simulink model "untitled3"  (Simulink 7.7)
settings: Solver=ode45  StartTime=0.0  StopTime=10.0  RelTol=1e-3
settings Model: Creator=güler  LastModifiedBy=güler

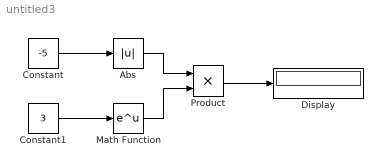
== system untitled3 ==
  Abs : Abs
  Constant : Constant  Value=-5
  Constant1 : Constant  Value=3
  Display : Display
  Math Function : Math  SaturateOnIntegerOverflow=on
  Product : Product  RndMeth=Zero
  wires:
  Product/1 -> Display/1
  Constant/1 -> Abs/1
  Constant1/1 -> Math Function/1
  Math Function/1 -> Product/2
  Abs/1 -> Product/1
